simulink model "gm_ModeS_ADI_Codegen"  (R2017a)
settings: Solver=VariableStepDiscrete  StartTime=0.0  StopTime=1e6  RelTol=1e-3
PreLoadFcn:
  | load data_Yb;
  | 
  | DataIn = Yb_with_time(:,2);
  | 
  | wl=16;
undefined symbols (not defined in the file or in its folder): dfilt
libraries: simulink x3, dspobslib x2, dspsnks4 x2, hdlsllib x1, dspindex x1, dspsrcs4 x1
settings Model: Creator=mdonovan  LastModifiedBy=ACozma
settings DataIOCC: LimitDataPoints=on  SaveFormat=Array  SignalLoggingSaveFormat=ModelDataLogs  SaveOutput=off  SignalLogging=off  SaveTime=off
settings OptimizationCC: BlockReduction=off  BooleanDataType=off  ConditionallyExecuteInputs=off  DefaultParameterBehavior=Inlined  ExpressionDepthLimit=2147483647  LocalBlockOutputs=off  LifeSpan=inf
settings DebuggingCC: AlgebraicLoopMsg=error  UnderspecifiedInitializationDetection=Classic  MergeDetectMultiDrivingBlocksExec=none  SolverPrmCheckMsg=warning  InheritedTsInSrcMsg=none  SingleTaskRateTransMsg=error  FcnCallInpInsideContextMsg=warning  AllowSymbolicDim=off  StateNameClashWarn=warning  SFUnexpectedBacktrackingDiag=warning  SFNoUnconditionalDefaultTransitionDiag=warning  SFExecutionAtInitializationDiag=none
settings HardwareCC: ProdBitPerPointer=32  ProdBitPerSizeT=32  ProdBitPerPtrDiffT=32  ProdLargestAtomicFloat=None  ProdIntDivRoundTo=Undefined  ProdEndianess=Unspecified  ProdWordSize=32  ProdHWDeviceType=ASIC/FPGA->ASIC/FPGA  TargetBitPerPointer=64  TargetBitPerSizeT=64  TargetBitPerPtrDiffT=64  TargetLongLongMode=on  TargetIntDivRoundTo=Zero  TargetEndianess=LittleEndian  TargetWordSize=64  TargetHWDeviceType=MATLAB Host  ProdEqTarget=off
settings ModelReferenceCC: PropagateSignalLabelsOutOfModel=off
settings GRTTargetCC: TargetLangStandard=C89/C90 (ANSI)  GeneratePreprocessorConditionals=Disable all  CombineOutputUpdateFcns=off  GRTInterface=on
settings ConfigComp: CovMetricSettings=dw  CovHtmlReporting=on  CovSaveCumulativeToWorkspaceVar=on  CovSaveSingleToWorkspaceVar=on  CovExternalEMLEnable=off

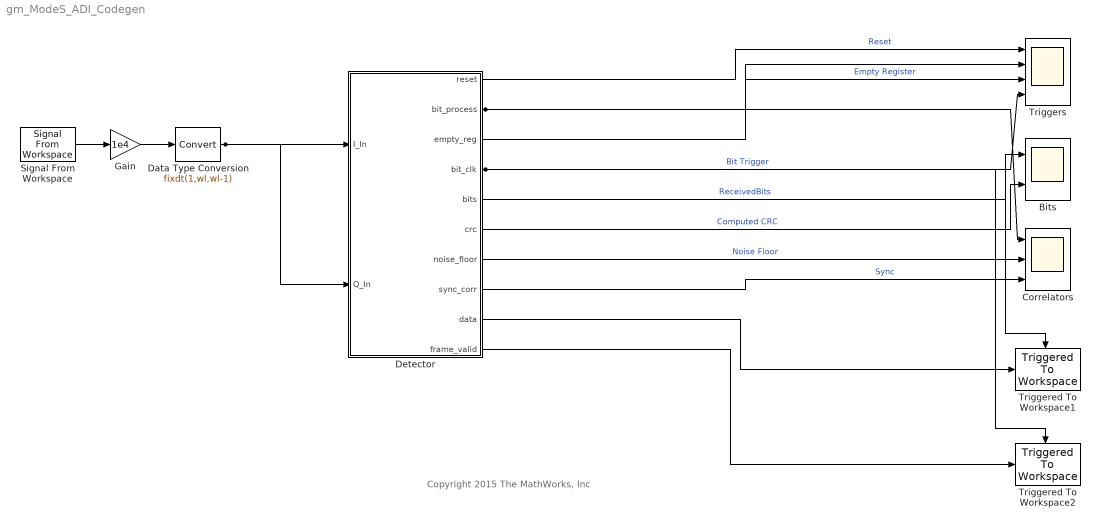
== system gm_ModeS_ADI_Codegen ==
  note: Copyright 2015 The MathWorks, Inc
  Bits : Scope  NumInputPorts=2
  Correlators : Scope  NumInputPorts=3
  Data Type Conversion : DataTypeConversion  OutDataTypeStr=fixdt(1,wl,wl-1)  LockScale=on
  Detector : Subsystem  TreatAsAtomicUnit=on
  Gain : Gain  Gain=1e4
  Signal From Workspace : dspsrcs4/Signal From Workspace  X=DataIn  Ts=1  nsamps=1  OutputAfterFinalValue=Setting to zero  ignoreOrWarnInputAndFrameLengths=off  OutputFrames=on
  Triggered To Workspace1 : dspsnks4/Triggered To Workspace  TriggerType=Rising edge  VariableName=data_out  Buffer=1000  Save2DMode=2-D array (concatenate along first dimension)
      settings: SourceProductName=DSP System Toolbox  SourceProductBaseCode=DS  FixptAsFi=off
  Triggered To Workspace2 : dspsnks4/Triggered To Workspace  TriggerType=Rising edge  VariableName=frame_valid  Buffer=1000  Save2DMode=2-D array (concatenate along first dimension)
      settings: SourceProductName=DSP System Toolbox  SourceProductBaseCode=DS  FixptAsFi=off
  Triggers : Scope  NumInputPorts=4
  wires:
  Detector/8(sync_corr) -> Correlators/3  "Sync"
  Detector/3(empty_reg) -> Triggers/3  "Empty Register"
  Detector/2(bit_process) -> Correlators/1, Triggers/2
  Detector/1(reset) -> Triggers/1  "Reset"
  Detector/6(crc) -> Bits/2  "Computed CRC"
  Detector/7(noise_floor) -> Correlators/2  "Noise Floor"
  Detector/9(data) -> Triggered To Workspace1/1
  Detector/10(frame_valid) -> Triggered To Workspace2/1
  Detector/4(bit_clk) -> Triggers/4, Triggered To Workspace1/Trigger, Triggered To Workspace2/Trigger  "Bit Trigger"
  Detector/5(bits) -> Bits/1  "ReceivedBits"
  Gain/1 -> Data Type Conversion/1
  Data Type Conversion/1 -> Detector/2(Q_In), Detector/1(I_In)
  Signal From Workspace/1 -> Gain/1

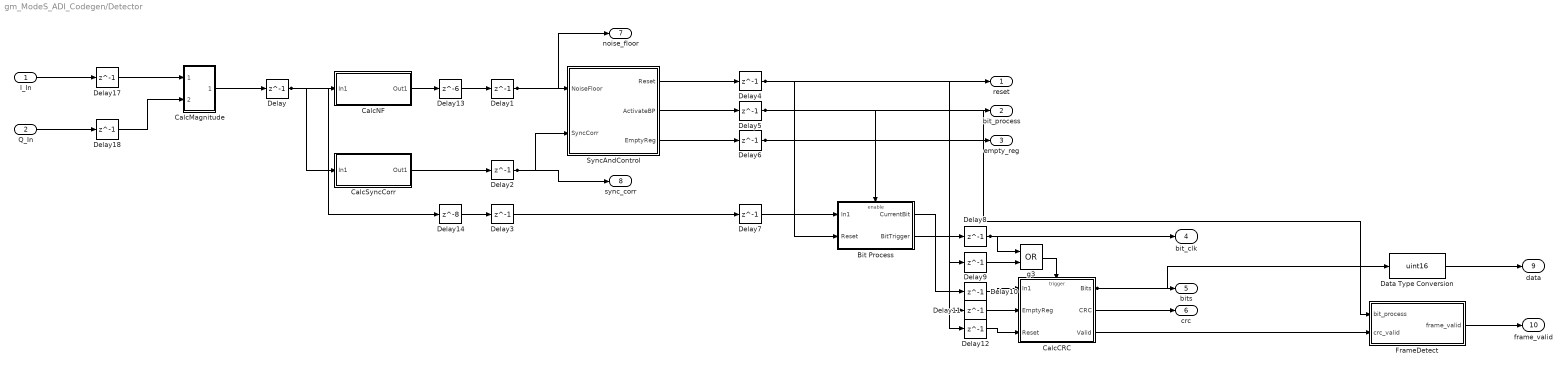
== system gm_ModeS_ADI_Codegen/Detector ==
  I_In : Inport  OutDataTypeStr=fixdt(1, 16, 15)  SampleTime=1
  Q_In : Inport  Port=2  OutDataTypeStr=fixdt(1, 16, 15)  SampleTime=1
  Bit Process : Subsystem
  CalcCRC : Subsystem
  CalcMagnitude : Subsystem
  CalcNF : Subsystem
  CalcSyncCorr : Subsystem
  Data Type Conversion : DataTypeConversion  OutDataTypeStr=uint16
  Delay{,1..12,17..18} (15 alike) : Delay  DelayLength=1  InitialCondition=0  InputProcessing=Columns as channels (frame based)
  Delay13 : Delay  DelayLength=6  InitialCondition=0  InputProcessing=Columns as channels (frame based)
  Delay14 : Delay  DelayLength=8  InitialCondition=0  InputProcessing=Columns as channels (frame based)
  FrameDetect : Subsystem
  SyncAndControl : Subsystem
  g3 : Logic  Operator=OR  AllPortsSameDT=off  OutDataTypeStr=boolean
  reset : Outport
  bit_process : Outport  Port=2
  empty_reg : Outport  Port=3
  bit_clk : Outport  Port=4
  bits : Outport  Port=5
  crc : Outport  Port=6
  noise_floor : Outport  Port=7
  sync_corr : Outport  Port=8
  data : Outport  Port=9
  frame_valid : Outport  Port=10
  wires:
  I_In/1 -> Delay17/1
  Q_In/1 -> Delay18/1
  Bit Process/1(CurrentBit) -> Delay10/1
  Bit Process/2(BitTrigger) -> Delay8/1
  CalcCRC/1(Bits) -> Data Type Conversion/1, bits/1
  CalcCRC/2(CRC) -> crc/1
  CalcCRC/3(Valid) -> FrameDetect/2(crc_valid)
  CalcMagnitude/1(Out1) -> Delay/1
  CalcNF/1(Out1) -> Delay13/1
  CalcSyncCorr/1(Out1) -> Delay2/1
  Data Type Conversion/1 -> data/1
  Delay/1 -> Delay14/1, CalcNF/1(In1), CalcSyncCorr/1(In1)
  Delay1/1 -> SyncAndControl/1(NoiseFloor), noise_floor/1
  Delay10/1 -> CalcCRC/1(In1)
  Delay11/1 -> CalcCRC/2(EmptyReg)
  Delay12/1 -> CalcCRC/3(Reset)
  Delay13/1 -> Delay1/1
  Delay14/1 -> Delay3/1
  Delay17/1 -> CalcMagnitude/1(In1)
  Delay18/1 -> CalcMagnitude/2(In2)
  Delay2/1 -> SyncAndControl/2(SyncCorr), sync_corr/1
  Delay3/1 -> Delay7/1
  Delay4/1 -> Delay9/1, Delay12/1, reset/1, Bit Process/2(Reset)
  Delay5/1 -> FrameDetect/1(bit_process), Bit Process/Enable, bit_process/1
  Delay6/1 -> Delay11/1, empty_reg/1
  Delay7/1 -> Bit Process/1(In1)
  Delay8/1 -> g3/1, bit_clk/1
  Delay9/1 -> g3/2
  FrameDetect/1(frame_valid) -> frame_valid/1
  SyncAndControl/1(Reset) -> Delay4/1
  SyncAndControl/2(ActivateBP) -> Delay5/1
  SyncAndControl/3(EmptyReg) -> Delay6/1
  g3/1 -> CalcCRC/Trigger

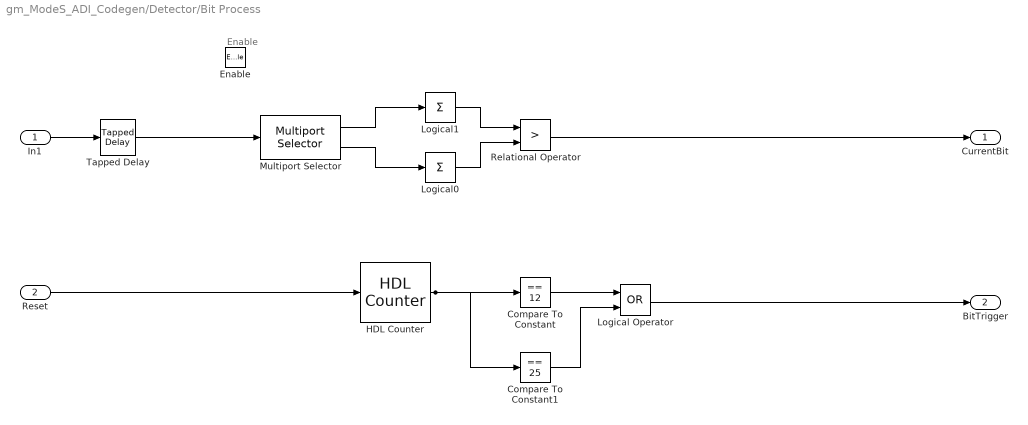
== system gm_ModeS_ADI_Codegen/Detector/Bit Process ==
  note: Enable
  In1 : Inport  SampleTime=1
  Reset : Inport  Port=2  SampleTime=1
  Enable : EnablePort
  Compare To Constant : simulink/Logic and Bit Operations/Compare To Constant  relop===  const=12  OutDataTypeStr=boolean
  Compare To Constant1 : simulink/Logic and Bit Operations/Compare To Constant  relop===  const=25  OutDataTypeStr=boolean
  HDL Counter : hdlsllib/HDL Operations/HDL Counter  CountType=Count limited  CountInit=1  CountStep=1  CountMax=25  CountFromType=Initial value  CountFrom=1  CountResetPort=on  CountLoadPort=off  CountEnbPort=off  CountDirPort=off  CountDataType=Unsigned  CountWordLen=8  CountFracLen=0  CountSampTime=1
      settings: SourceProductName=HDL Coder  SourceProductBaseCode=HD
  Logical Operator : Logic  Operator=OR  AllPortsSameDT=off  OutDataTypeStr=boolean
  Logical0 : Sum  Inputs=+  AccumDataTypeStr=fixdt(1,wl,wl-3)  OutDataTypeStr=Inherit: Same as accumulator
  Logical1 : Sum  Inputs=+  AccumDataTypeStr=fixdt(1,wl,wl-3)  OutDataTypeStr=Inherit: Same as accumulator
  Multiport Selector : dspindex/Multiport Selector  rowsOrCols=Rows  idxCellArray={ 1:6,7:12}  idxErrMode=Clip Index
  Relational Operator : RelationalOperator  Operator=>  OutDataTypeStr=boolean  RndMeth=Nearest
  Tapped Delay : simulink/Discrete/Tapped Delay  vinit=0.0  samptime=1  NumDelays=12  DelayOrder=Oldest  includeCurrent=on
  CurrentBit : Outport  InitialOutput=0
  BitTrigger : Outport  Port=2  InitialOutput=0
  wires:
  In1/1 -> Tapped Delay/1
  Reset/1 -> HDL Counter/1
  Compare To Constant/1 -> Logical Operator/1
  Compare To Constant1/1 -> Logical Operator/2
  HDL Counter/1 -> Compare To Constant1/1, Compare To Constant/1
  Logical Operator/1 -> BitTrigger/1
  Logical0/1 -> Relational Operator/2
  Logical1/1 -> Relational Operator/1
  Multiport Selector/1 -> Logical1/1
  Multiport Selector/2 -> Logical0/1
  Relational Operator/1 -> CurrentBit/1
  Tapped Delay/1 -> Multiport Selector/1

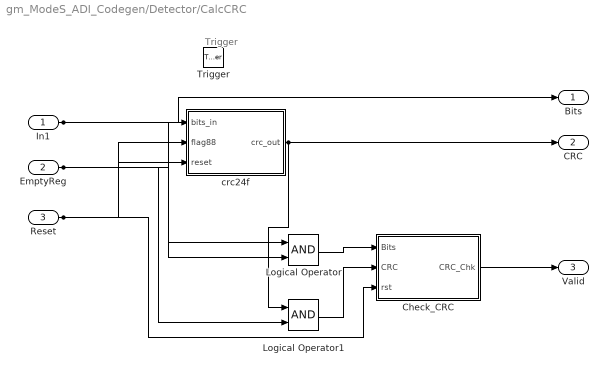
== system gm_ModeS_ADI_Codegen/Detector/CalcCRC ==
  note: Trigger
  In1 : Inport
  EmptyReg : Inport  Port=2
  Reset : Inport  Port=3
  Trigger : TriggerPort  VariantControl=Variant
  Check_CRC : Subsystem
  Logical Operator : Logic  AllPortsSameDT=off  OutDataTypeStr=boolean
  Logical Operator1 : Logic  AllPortsSameDT=off  OutDataTypeStr=boolean
  crc24f : Subsystem
  Bits : Outport  InitialOutput=0
  CRC : Outport  Port=2  InitialOutput=0
  Valid : Outport  Port=3  InitialOutput=0
  wires:
  In1/1 -> Logical Operator/1, Bits/1, crc24f/1(bits_in)
  EmptyReg/1 -> Logical Operator1/2, Logical Operator/2, crc24f/2(flag88)
  Reset/1 -> Check_CRC/3(rst), crc24f/3(reset)
  Check_CRC/1(CRC_Chk) -> Valid/1
  Logical Operator/1 -> Check_CRC/1(Bits)
  Logical Operator1/1 -> Check_CRC/2(CRC)
  crc24f/1(crc_out) -> Logical Operator1/1, CRC/1

== system gm_ModeS_ADI_Codegen/Detector/CalcMagnitude ==
  In1 : Inport  SampleTime=1
  In2 : Inport  Port=2  SampleTime=1
  Add : Sum  OutDataTypeStr=fixdt(1,wl,wl-1)
  Delay15 : Delay  DelayLength=1  InitialCondition=0  InputProcessing=Columns as channels (frame based)
  Delay16 : Delay  DelayLength=1  InitialCondition=0  InputProcessing=Columns as channels (frame based)
  Product : Product  OutDataTypeStr=fixdt(1,wl,wl-1)
  Product1 : Product  OutDataTypeStr=fixdt(1,wl,wl-1)
  Out1 : Outport
  wires:
  In1/1 -> Product/2, Product/1
  In2/1 -> Product1/2, Product1/1
  Add/1 -> Out1/1
  Delay15/1 -> Add/1
  Delay16/1 -> Add/2
  Product/1 -> Delay15/1
  Product1/1 -> Delay16/1

== system gm_ModeS_ADI_Codegen/Detector/CalcNF ==
  In1 : Inport  SampleTime=1
  NoiseFloor : Subsystem
      settings: DeleteFcn=dspLinkFVTool2Mask(gcbh,'close')  ModelCloseFcn=dspLinkFVTool2Mask(gcbh,'close')  CloseFcn=dspLinkFVTool2Mask(gcbh,'close')
  Out1 : Outport
  wires:
  In1/1 -> NoiseFloor/1(In1)
  NoiseFloor/1(Out1) -> Out1/1

== system gm_ModeS_ADI_Codegen/Detector/CalcSyncCorr ==
  In1 : Inport  SampleTime=1
  SyncCorr : Subsystem
      settings: DeleteFcn=dspLinkFVTool2Mask(gcbh,'close')  ModelCloseFcn=dspLinkFVTool2Mask(gcbh,'close')  CloseFcn=dspLinkFVTool2Mask(gcbh,'close')
  Out1 : Outport
  wires:
  In1/1 -> SyncCorr/1(In1)
  SyncCorr/1(Out1) -> Out1/1

== system gm_ModeS_ADI_Codegen/Detector/FrameDetect ==
  bit_process : Inport  SampleTime=1
  crc_valid : Inport  Port=2  SampleTime=1
  Data Type Conversion : DataTypeConversion  OutDataTypeStr=uint16
  Delay14 : Delay  DelayLength=1  InitialCondition=0  InputProcessing=Columns as channels (frame based)
  Logical Operator : Logic  AllPortsSameDT=off  OutDataTypeStr=boolean
  Logical Operator1 : Logic  Operator=NOT  AllPortsSameDT=off  OutDataTypeStr=boolean
  Logical Operator2 : Logic  AllPortsSameDT=off  OutDataTypeStr=boolean
  frame_valid : Outport
  wires:
  bit_process/1 -> Logical Operator1/1, Delay14/1
  crc_valid/1 -> Logical Operator2/1
  Data Type Conversion/1 -> frame_valid/1
  Delay14/1 -> Logical Operator/2
  Logical Operator/1 -> Logical Operator2/2
  Logical Operator1/1 -> Logical Operator/1
  Logical Operator2/1 -> Data Type Conversion/1

== system gm_ModeS_ADI_Codegen/Detector/SyncAndControl ==
  NoiseFloor : Inport  SampleTime=1
  SyncCorr : Inport  Port=2  SampleTime=1
  SyncAndControl : Stateflow chart  TreatAsAtomicUnit=on
  Reset : Outport
  ActivateBP : Outport  Port=2
  EmptyReg : Outport  Port=3
  wires:
  NoiseFloor/1 -> SyncAndControl/1(NoiseFloor)
  SyncCorr/1 -> SyncAndControl/2(SyncCorr)
  SyncAndControl/1(Reset) -> Reset/1
  SyncAndControl/2(ActivateBP) -> ActivateBP/1
  SyncAndControl/3(EmptyReg) -> EmptyReg/1

== system gm_ModeS_ADI_Codegen/Detector/CalcCRC/Check_CRC ==
  note: Remember any difference
  note: Comparison
  Bits : Inport
  CRC : Inport  Port=2
  rst : Inport  Port=3
  Delay : Delay  DelayLength=1  ExternalReset=Level
      settings: InputPortMap=u0,r5
  Logical Operator : Logic  Operator=XOR  AllPortsSameDT=off  OutDataTypeStr=boolean
  Logical Operator1 : Logic  Operator=OR  AllPortsSameDT=off  OutDataTypeStr=boolean
  Logical Operator2 : Logic  Operator=NOT  AllPortsSameDT=off  OutDataTypeStr=boolean
  CRC_Chk : Outport  InitialOutput=0
  wires:
  Bits/1 -> Logical Operator/1
  CRC/1 -> Logical Operator/2
  rst/1 -> Delay/2
  Logical Operator/1 -> Logical Operator1/1
  Logical Operator1/1 -> Logical Operator2/1, Delay/1
  Logical Operator2/1 -> CRC_Chk/1
  Delay/1 -> Logical Operator1/2

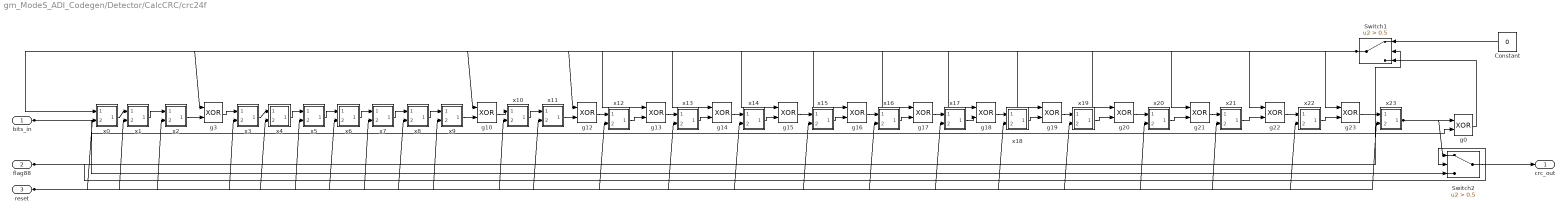
== system gm_ModeS_ADI_Codegen/Detector/CalcCRC/crc24f ==
  bits_in : Inport
  flag88 : Inport  Port=2
  reset : Inport  Port=3
  Constant : Constant  Value=0  OutDataTypeStr=boolean  SampleTime=-1
  Switch1 : Switch  Criteria=u2 > Threshold  Threshold=0.5
  Switch2 : Switch  Criteria=u2 > Threshold  Threshold=0.5
  g{0,3,10,12..23} (15 alike) : Logic  Operator=XOR  AllPortsSameDT=off  OutDataTypeStr=boolean
  x0 : Subsystem
  x1 : Subsystem
  x10 : Subsystem
  x11 : Subsystem
  x12 : Subsystem
  x13 : Subsystem
  x14 : Subsystem
  x15 : Subsystem
  x16 : Subsystem
  x17 : Subsystem
  x18 : Subsystem
  x19 : Subsystem
  x2 : Subsystem
  x20 : Subsystem
  x21 : Subsystem
  x22 : Subsystem
  x23 : Subsystem
  x3 : Subsystem
  x4 : Subsystem
  x5 : Subsystem
  x6 : Subsystem
  x7 : Subsystem
  x8 : Subsystem
  x9 : Subsystem
  crc_out : Outport  InitialOutput=0
  wires:
  bits_in/1 -> Switch2/3, g0/2
  flag88/1 -> Switch2/2, Switch1/2
  reset/1 -> x0/2(Reset), x1/2(Reset), x10/2(Reset), x11/2(Reset), x12/2(Reset), x13/2(Reset), x14/2(Reset), x15/2(Reset), x16/2(Reset), x17/2(Reset), x18/2(Reset), x19/2(Reset), x2/2(Reset), x20/2(Reset), x21/2(Reset), x22/2(Reset), x23/2(Reset), x3/2(Reset), x4/2(Reset), x5/2(Reset), x6/2(Reset), x7/2(Reset), x8/2(Reset), x9/2(Reset)
  Constant/1 -> Switch1/1
  Switch2/1 -> crc_out/1
  x23/1(data_out) -> Switch2/1, g0/1
  x22/1(data_out) -> g23/2
  g22/1 -> x22/1(data_in)
  x21/1(data_out) -> g22/2
  g21/1 -> x21/1(data_in)
  x20/1(data_out) -> g21/2
  g20/1 -> x20/1(data_in)
  x19/1(data_out) -> g20/2
  g19/1 -> x19/1(data_in)
  x18/1(data_out) -> g19/2
  g18/1 -> x18/1(data_in)
  x17/1(data_out) -> g18/2
  g17/1 -> x17/1(data_in)
  x16/1(data_out) -> g17/2
  g16/1 -> x16/1(data_in)
  x15/1(data_out) -> g16/2
  g15/1 -> x15/1(data_in)
  x14/1(data_out) -> g15/2
  g14/1 -> x14/1(data_in)
  x13/1(data_out) -> g14/2
  g13/1 -> x13/1(data_in)
  x12/1(data_out) -> g13/2
  g12/1 -> x12/1(data_in)
  x11/1(data_out) -> g12/2
  x10/1(data_out) -> x11/1(data_in)
  g10/1 -> x10/1(data_in)
  x9/1(data_out) -> g10/2
  x8/1(data_out) -> x9/1(data_in)
  x7/1(data_out) -> x8/1(data_in)
  x6/1(data_out) -> x7/1(data_in)
  x5/1(data_out) -> x6/1(data_in)
  x4/1(data_out) -> x5/1(data_in)
  x3/1(data_out) -> x4/1(data_in)
  g3/1 -> x3/1(data_in)
  x2/1(data_out) -> g3/2
  x1/1(data_out) -> x2/1(data_in)
  x0/1(data_out) -> x1/1(data_in)
  g0/1 -> Switch1/3
  Switch1/1 -> g3/1, g23/1, g22/1, g21/1, g20/1, g19/1, g18/1, g17/1, g16/1, g15/1, g14/1, g13/1, g12/1, g10/1, x0/1(data_in)
  g23/1 -> x23/1(data_in)

== system gm_ModeS_ADI_Codegen/Detector/CalcNF/NoiseFloor ==
  In1 : Inport
  NoiseFloor : dspobslib/Digital Filter  TypePopup=FIR (all zeros)  IIRFiltStruct=Direct form II transposed  AllPoleFiltStruct=Direct form  FIRFiltStruct=Direct form transposed  CoeffSource=Specify via dialog  NumCoeffs=(ones(64,1)/64)  DenCoeffs=[1 0.1]  BiQuadCoeffs=[1 0.3 0.4 1 0.1 0.2]  LatticeCoeffs=[0.2 0.4]  denIgnore=on  FiltPerSampPopup=One filter per frame  IC=0  ICnum=0  ICden=0  firstCoeffMode=Binary point scaling  firstCoeffWordLength=wl  firstCoeffFracLength=wl+4  outputMode=Binary point scaling  outputWordLength=wl  outputFracLength=wl  accumMode=Binary point scaling  accumWordLength=wl*2  accumFracLength=wl*2  prodOutputMode=Binary point scaling  prodOutputWordLength=wl*2  prodOutputFracLength=wl*2+5  roundingMode=Floor  overflowMode=off  ScaleValues=1  scaleValueFracLength=14  stageInFracLength=15  stageOutFracLength=15  FilterSource=Specify via dialog  dfiltObjectName=dfilt.dffir([1 2 1])  InputProcessing=Columns as channels (frame based)
      settings: SourceProductName=DSP System Toolbox  SourceProductBaseCode=DS
  NoiseFloor_GenDelay1 : Delay  InputProcessing=Inherited
  Out1 : Outport
  wires:
  In1/1 -> NoiseFloor/1
  NoiseFloor/1 -> NoiseFloor_GenDelay1/1
  NoiseFloor_GenDelay1/1 -> Out1/1

== system gm_ModeS_ADI_Codegen/Detector/CalcSyncCorr/SyncCorr ==
  In1 : Inport
  SyncCorr : dspobslib/Digital Filter  TypePopup=FIR (all zeros)  IIRFiltStruct=Direct form II transposed  AllPoleFiltStruct=Direct form  FIRFiltStruct=Direct form  CoeffSource=Specify via dialog  NumCoeffs=|  DenCoeffs=[1 0.1]  BiQuadCoeffs=[1 0.3 0.4 1 0.1 0.2]  LatticeCoeffs=[0.2 0.4]  denIgnore=on  FiltPerSampPopup=One filter per frame  IC=0  ICnum=0  ICden=0  firstCoeffMode=Binary point scaling  firstCoeffWordLength=16  firstCoeffFracLength=14  outputMode=Binary point scaling  outputWordLength=16  outputFracLength=11  accumMode=Binary point scaling  accumWordLength=37  accumFracLength=29  prodOutputMode=Binary point scaling  prodOutputWordLength=31  prodOutputFracLength=29  roundingMode=Floor  overflowMode=off  ScaleValues=1  scaleValueFracLength=14  stageInFracLength=15  stageOutFracLength=15  FilterSource=Specify via dialog  dfiltObjectName=dfilt.dffir([1 2 1])  InputProcessing=Columns as channels (frame based)
      | flipud([ones(6,1);-1*ones(6,1);ones(6,1);-1*ones(7,1);
      | -1*ones(6,1);-1*ones(6,1);-1*ones(6,1);ones(7,1);-1*ones(6,1);ones(6,1);-1*ones(6,1);-1*ones(7,1)])
      settings: SourceProductName=DSP System Toolbox  SourceProductBaseCode=DS
  SyncCorr_GenDelay1 : Delay  DelayLength=8  InputProcessing=Inherited
  Out1 : Outport
  wires:
  In1/1 -> SyncCorr/1
  SyncCorr/1 -> SyncCorr_GenDelay1/1
  SyncCorr_GenDelay1/1 -> Out1/1

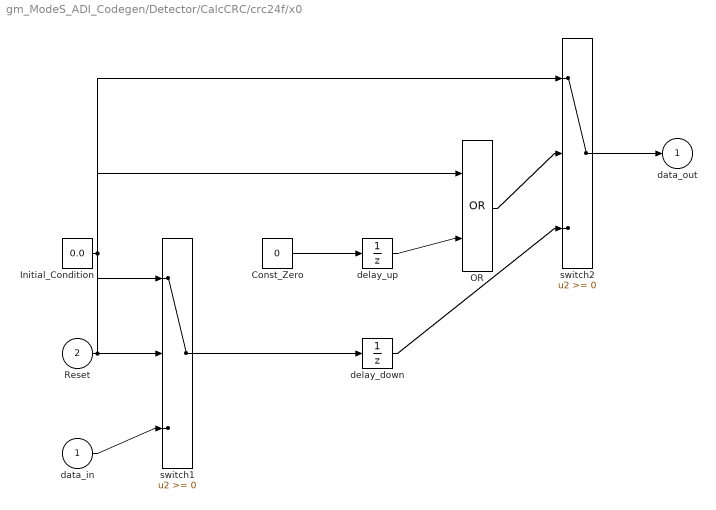
== system gm_ModeS_ADI_Codegen/Detector/CalcCRC/crc24f/x0 ==
  data_in : Inport
  Reset : Inport  Port=2
  Const_Zero : Constant  Value=0  OutDataTypeStr=boolean
  Initial_Condition : Constant  Value=0.0  OutDataTypeStr=Inherit: Inherit via back propagation
  OR : Logic  Operator=OR
  delay_down : UnitDelay  SampleTime=-1
  delay_up : UnitDelay  InitialCondition=1  SampleTime=-1
  switch1 : Switch  SaturateOnIntegerOverflow=on  InputSameDT=on
  switch2 : Switch  SaturateOnIntegerOverflow=on  InputSameDT=on
  data_out : Outport
  wires:
  Initial_Condition/1 -> switch1/1, switch2/1
  Reset/1 -> switch1/2, OR/1
  data_in/1 -> switch1/3
  Const_Zero/1 -> delay_up/1
  switch1/1 -> delay_down/1
  delay_up/1 -> OR/2
  OR/1 -> switch2/2
  delay_down/1 -> switch2/3
  switch2/1 -> data_out/1

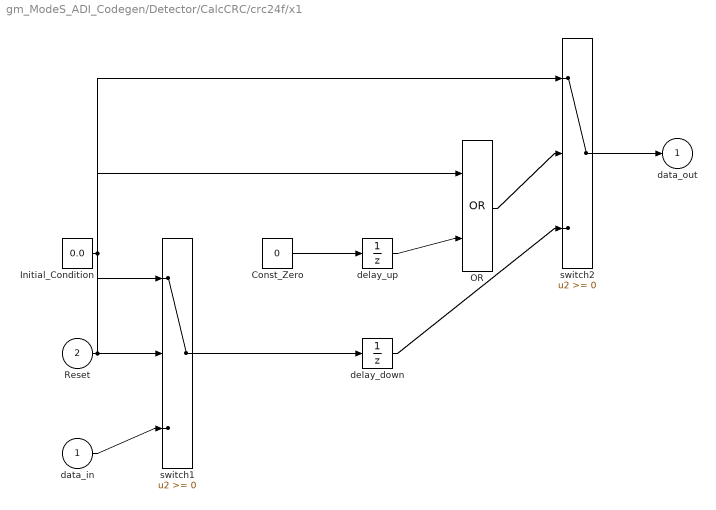
== system gm_ModeS_ADI_Codegen/Detector/CalcCRC/crc24f/x1 ==
  data_in : Inport
  Reset : Inport  Port=2
  Const_Zero : Constant  Value=0  OutDataTypeStr=boolean
  Initial_Condition : Constant  Value=0.0  OutDataTypeStr=Inherit: Inherit via back propagation
  OR : Logic  Operator=OR
  delay_down : UnitDelay  SampleTime=-1
  delay_up : UnitDelay  InitialCondition=1  SampleTime=-1
  switch1 : Switch  SaturateOnIntegerOverflow=on  InputSameDT=on
  switch2 : Switch  SaturateOnIntegerOverflow=on  InputSameDT=on
  data_out : Outport
  wires:
  Initial_Condition/1 -> switch1/1, switch2/1
  Reset/1 -> switch1/2, OR/1
  data_in/1 -> switch1/3
  Const_Zero/1 -> delay_up/1
  switch1/1 -> delay_down/1
  delay_up/1 -> OR/2
  OR/1 -> switch2/2
  delay_down/1 -> switch2/3
  switch2/1 -> data_out/1

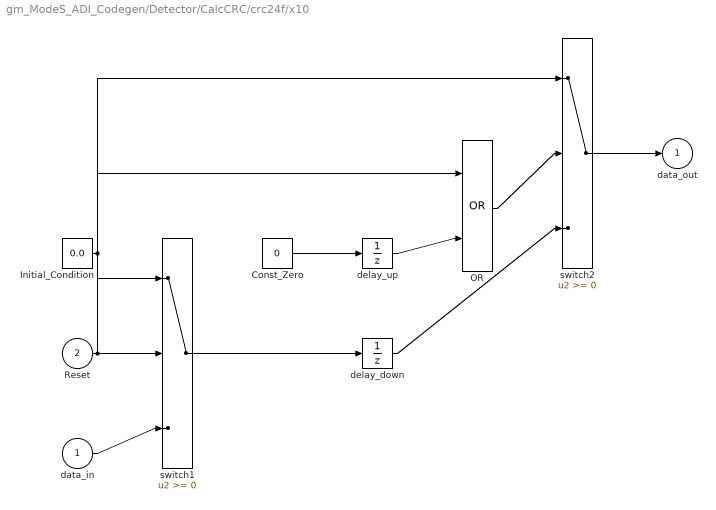
== system gm_ModeS_ADI_Codegen/Detector/CalcCRC/crc24f/x10 ==
  data_in : Inport
  Reset : Inport  Port=2
  Const_Zero : Constant  Value=0  OutDataTypeStr=boolean
  Initial_Condition : Constant  Value=0.0  OutDataTypeStr=Inherit: Inherit via back propagation
  OR : Logic  Operator=OR
  delay_down : UnitDelay  SampleTime=-1
  delay_up : UnitDelay  InitialCondition=1  SampleTime=-1
  switch1 : Switch  SaturateOnIntegerOverflow=on  InputSameDT=on
  switch2 : Switch  SaturateOnIntegerOverflow=on  InputSameDT=on
  data_out : Outport
  wires:
  Initial_Condition/1 -> switch1/1, switch2/1
  Reset/1 -> switch1/2, OR/1
  data_in/1 -> switch1/3
  Const_Zero/1 -> delay_up/1
  switch1/1 -> delay_down/1
  delay_up/1 -> OR/2
  OR/1 -> switch2/2
  delay_down/1 -> switch2/3
  switch2/1 -> data_out/1

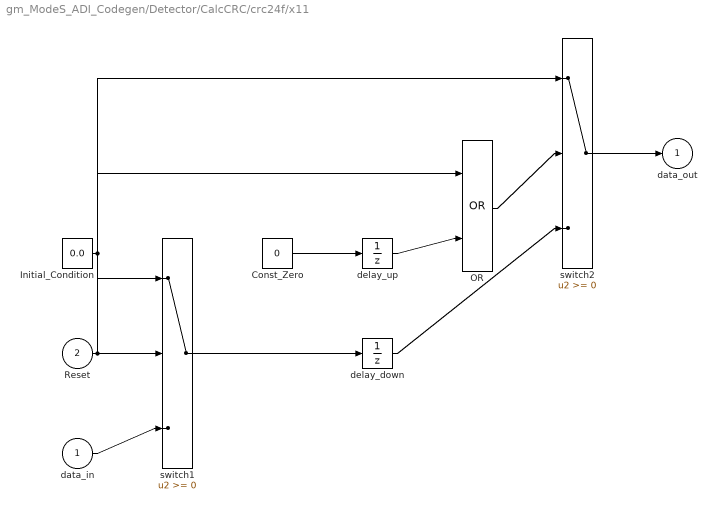
== system gm_ModeS_ADI_Codegen/Detector/CalcCRC/crc24f/x11 ==
  data_in : Inport
  Reset : Inport  Port=2
  Const_Zero : Constant  Value=0  OutDataTypeStr=boolean
  Initial_Condition : Constant  Value=0.0  OutDataTypeStr=Inherit: Inherit via back propagation
  OR : Logic  Operator=OR
  delay_down : UnitDelay  SampleTime=-1
  delay_up : UnitDelay  InitialCondition=1  SampleTime=-1
  switch1 : Switch  SaturateOnIntegerOverflow=on  InputSameDT=on
  switch2 : Switch  SaturateOnIntegerOverflow=on  InputSameDT=on
  data_out : Outport
  wires:
  Initial_Condition/1 -> switch1/1, switch2/1
  Reset/1 -> switch1/2, OR/1
  data_in/1 -> switch1/3
  Const_Zero/1 -> delay_up/1
  switch1/1 -> delay_down/1
  delay_up/1 -> OR/2
  OR/1 -> switch2/2
  delay_down/1 -> switch2/3
  switch2/1 -> data_out/1

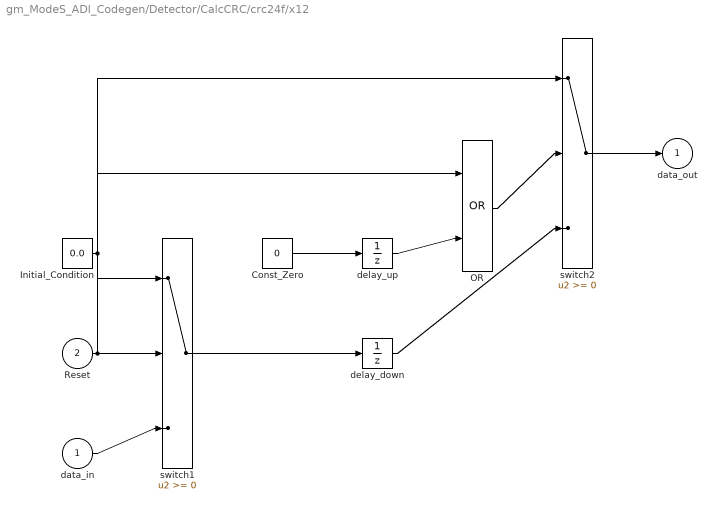
== system gm_ModeS_ADI_Codegen/Detector/CalcCRC/crc24f/x12 ==
  data_in : Inport
  Reset : Inport  Port=2
  Const_Zero : Constant  Value=0  OutDataTypeStr=boolean
  Initial_Condition : Constant  Value=0.0  OutDataTypeStr=Inherit: Inherit via back propagation
  OR : Logic  Operator=OR
  delay_down : UnitDelay  SampleTime=-1
  delay_up : UnitDelay  InitialCondition=1  SampleTime=-1
  switch1 : Switch  SaturateOnIntegerOverflow=on  InputSameDT=on
  switch2 : Switch  SaturateOnIntegerOverflow=on  InputSameDT=on
  data_out : Outport
  wires:
  Initial_Condition/1 -> switch1/1, switch2/1
  Reset/1 -> switch1/2, OR/1
  data_in/1 -> switch1/3
  Const_Zero/1 -> delay_up/1
  switch1/1 -> delay_down/1
  delay_up/1 -> OR/2
  OR/1 -> switch2/2
  delay_down/1 -> switch2/3
  switch2/1 -> data_out/1

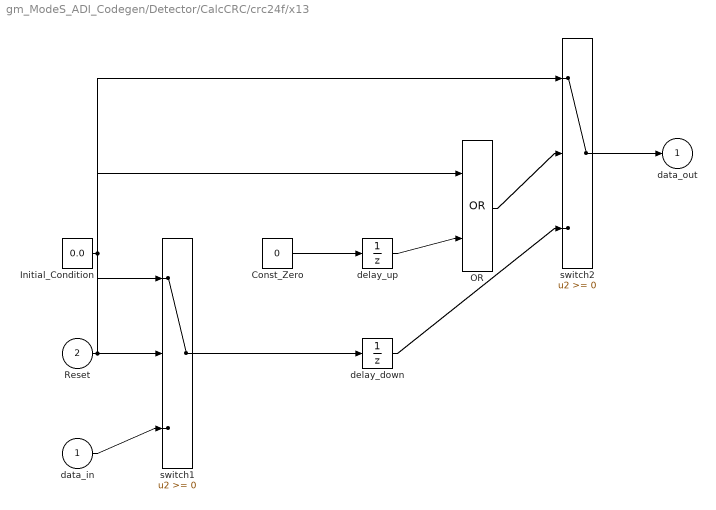
== system gm_ModeS_ADI_Codegen/Detector/CalcCRC/crc24f/x13 ==
  data_in : Inport
  Reset : Inport  Port=2
  Const_Zero : Constant  Value=0  OutDataTypeStr=boolean
  Initial_Condition : Constant  Value=0.0  OutDataTypeStr=Inherit: Inherit via back propagation
  OR : Logic  Operator=OR
  delay_down : UnitDelay  SampleTime=-1
  delay_up : UnitDelay  InitialCondition=1  SampleTime=-1
  switch1 : Switch  SaturateOnIntegerOverflow=on  InputSameDT=on
  switch2 : Switch  SaturateOnIntegerOverflow=on  InputSameDT=on
  data_out : Outport
  wires:
  Initial_Condition/1 -> switch1/1, switch2/1
  Reset/1 -> switch1/2, OR/1
  data_in/1 -> switch1/3
  Const_Zero/1 -> delay_up/1
  switch1/1 -> delay_down/1
  delay_up/1 -> OR/2
  OR/1 -> switch2/2
  delay_down/1 -> switch2/3
  switch2/1 -> data_out/1

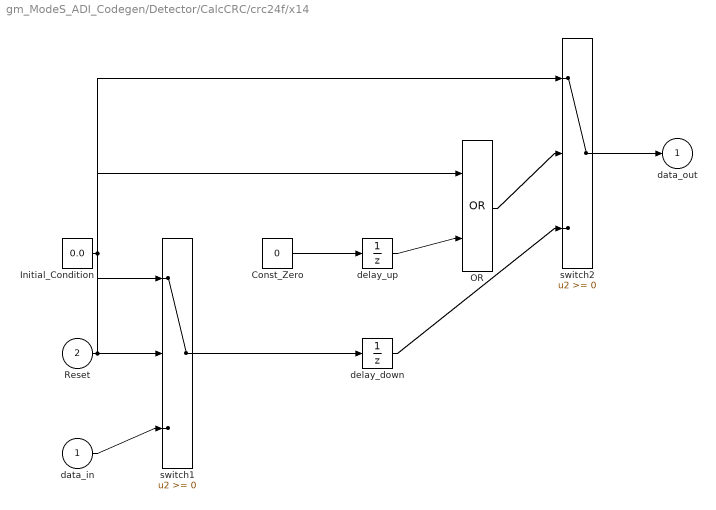
== system gm_ModeS_ADI_Codegen/Detector/CalcCRC/crc24f/x14 ==
  data_in : Inport
  Reset : Inport  Port=2
  Const_Zero : Constant  Value=0  OutDataTypeStr=boolean
  Initial_Condition : Constant  Value=0.0  OutDataTypeStr=Inherit: Inherit via back propagation
  OR : Logic  Operator=OR
  delay_down : UnitDelay  SampleTime=-1
  delay_up : UnitDelay  InitialCondition=1  SampleTime=-1
  switch1 : Switch  SaturateOnIntegerOverflow=on  InputSameDT=on
  switch2 : Switch  SaturateOnIntegerOverflow=on  InputSameDT=on
  data_out : Outport
  wires:
  Initial_Condition/1 -> switch1/1, switch2/1
  Reset/1 -> switch1/2, OR/1
  data_in/1 -> switch1/3
  Const_Zero/1 -> delay_up/1
  switch1/1 -> delay_down/1
  delay_up/1 -> OR/2
  OR/1 -> switch2/2
  delay_down/1 -> switch2/3
  switch2/1 -> data_out/1

== system gm_ModeS_ADI_Codegen/Detector/CalcCRC/crc24f/x15 ==
  data_in : Inport
  Reset : Inport  Port=2
  Const_Zero : Constant  Value=0  OutDataTypeStr=boolean
  Initial_Condition : Constant  Value=0.0  OutDataTypeStr=Inherit: Inherit via back propagation
  OR : Logic  Operator=OR
  delay_down : UnitDelay  SampleTime=-1
  delay_up : UnitDelay  InitialCondition=1  SampleTime=-1
  switch1 : Switch  SaturateOnIntegerOverflow=on  InputSameDT=on
  switch2 : Switch  SaturateOnIntegerOverflow=on  InputSameDT=on
  data_out : Outport
  wires:
  Initial_Condition/1 -> switch1/1, switch2/1
  Reset/1 -> switch1/2, OR/1
  data_in/1 -> switch1/3
  Const_Zero/1 -> delay_up/1
  switch1/1 -> delay_down/1
  delay_up/1 -> OR/2
  OR/1 -> switch2/2
  delay_down/1 -> switch2/3
  switch2/1 -> data_out/1

== system gm_ModeS_ADI_Codegen/Detector/CalcCRC/crc24f/x16 ==
  data_in : Inport
  Reset : Inport  Port=2
  Const_Zero : Constant  Value=0  OutDataTypeStr=boolean
  Initial_Condition : Constant  Value=0.0  OutDataTypeStr=Inherit: Inherit via back propagation
  OR : Logic  Operator=OR
  delay_down : UnitDelay  SampleTime=-1
  delay_up : UnitDelay  InitialCondition=1  SampleTime=-1
  switch1 : Switch  SaturateOnIntegerOverflow=on  InputSameDT=on
  switch2 : Switch  SaturateOnIntegerOverflow=on  InputSameDT=on
  data_out : Outport
  wires:
  Initial_Condition/1 -> switch1/1, switch2/1
  Reset/1 -> switch1/2, OR/1
  data_in/1 -> switch1/3
  Const_Zero/1 -> delay_up/1
  switch1/1 -> delay_down/1
  delay_up/1 -> OR/2
  OR/1 -> switch2/2
  delay_down/1 -> switch2/3
  switch2/1 -> data_out/1

== system gm_ModeS_ADI_Codegen/Detector/CalcCRC/crc24f/x17 ==
  data_in : Inport
  Reset : Inport  Port=2
  Const_Zero : Constant  Value=0  OutDataTypeStr=boolean
  Initial_Condition : Constant  Value=0.0  OutDataTypeStr=Inherit: Inherit via back propagation
  OR : Logic  Operator=OR
  delay_down : UnitDelay  SampleTime=-1
  delay_up : UnitDelay  InitialCondition=1  SampleTime=-1
  switch1 : Switch  SaturateOnIntegerOverflow=on  InputSameDT=on
  switch2 : Switch  SaturateOnIntegerOverflow=on  InputSameDT=on
  data_out : Outport
  wires:
  Initial_Condition/1 -> switch1/1, switch2/1
  Reset/1 -> switch1/2, OR/1
  data_in/1 -> switch1/3
  Const_Zero/1 -> delay_up/1
  switch1/1 -> delay_down/1
  delay_up/1 -> OR/2
  OR/1 -> switch2/2
  delay_down/1 -> switch2/3
  switch2/1 -> data_out/1

== system gm_ModeS_ADI_Codegen/Detector/CalcCRC/crc24f/x18 ==
  data_in : Inport
  Reset : Inport  Port=2
  Const_Zero : Constant  Value=0  OutDataTypeStr=boolean
  Initial_Condition : Constant  Value=0.0  OutDataTypeStr=Inherit: Inherit via back propagation
  OR : Logic  Operator=OR
  delay_down : UnitDelay  SampleTime=-1
  delay_up : UnitDelay  InitialCondition=1  SampleTime=-1
  switch1 : Switch  SaturateOnIntegerOverflow=on  InputSameDT=on
  switch2 : Switch  SaturateOnIntegerOverflow=on  InputSameDT=on
  data_out : Outport
  wires:
  Initial_Condition/1 -> switch1/1, switch2/1
  Reset/1 -> switch1/2, OR/1
  data_in/1 -> switch1/3
  Const_Zero/1 -> delay_up/1
  switch1/1 -> delay_down/1
  delay_up/1 -> OR/2
  OR/1 -> switch2/2
  delay_down/1 -> switch2/3
  switch2/1 -> data_out/1

== system gm_ModeS_ADI_Codegen/Detector/CalcCRC/crc24f/x19 ==
  data_in : Inport
  Reset : Inport  Port=2
  Const_Zero : Constant  Value=0  OutDataTypeStr=boolean
  Initial_Condition : Constant  Value=0.0  OutDataTypeStr=Inherit: Inherit via back propagation
  OR : Logic  Operator=OR
  delay_down : UnitDelay  SampleTime=-1
  delay_up : UnitDelay  InitialCondition=1  SampleTime=-1
  switch1 : Switch  SaturateOnIntegerOverflow=on  InputSameDT=on
  switch2 : Switch  SaturateOnIntegerOverflow=on  InputSameDT=on
  data_out : Outport
  wires:
  Initial_Condition/1 -> switch1/1, switch2/1
  Reset/1 -> switch1/2, OR/1
  data_in/1 -> switch1/3
  Const_Zero/1 -> delay_up/1
  switch1/1 -> delay_down/1
  delay_up/1 -> OR/2
  OR/1 -> switch2/2
  delay_down/1 -> switch2/3
  switch2/1 -> data_out/1

== system gm_ModeS_ADI_Codegen/Detector/CalcCRC/crc24f/x2 ==
  data_in : Inport
  Reset : Inport  Port=2
  Const_Zero : Constant  Value=0  OutDataTypeStr=boolean
  Initial_Condition : Constant  Value=0.0  OutDataTypeStr=Inherit: Inherit via back propagation
  OR : Logic  Operator=OR
  delay_down : UnitDelay  SampleTime=-1
  delay_up : UnitDelay  InitialCondition=1  SampleTime=-1
  switch1 : Switch  SaturateOnIntegerOverflow=on  InputSameDT=on
  switch2 : Switch  SaturateOnIntegerOverflow=on  InputSameDT=on
  data_out : Outport
  wires:
  Initial_Condition/1 -> switch1/1, switch2/1
  Reset/1 -> switch1/2, OR/1
  data_in/1 -> switch1/3
  Const_Zero/1 -> delay_up/1
  switch1/1 -> delay_down/1
  delay_up/1 -> OR/2
  OR/1 -> switch2/2
  delay_down/1 -> switch2/3
  switch2/1 -> data_out/1

== system gm_ModeS_ADI_Codegen/Detector/CalcCRC/crc24f/x20 ==
  data_in : Inport
  Reset : Inport  Port=2
  Const_Zero : Constant  Value=0  OutDataTypeStr=boolean
  Initial_Condition : Constant  Value=0.0  OutDataTypeStr=Inherit: Inherit via back propagation
  OR : Logic  Operator=OR
  delay_down : UnitDelay  SampleTime=-1
  delay_up : UnitDelay  InitialCondition=1  SampleTime=-1
  switch1 : Switch  SaturateOnIntegerOverflow=on  InputSameDT=on
  switch2 : Switch  SaturateOnIntegerOverflow=on  InputSameDT=on
  data_out : Outport
  wires:
  Initial_Condition/1 -> switch1/1, switch2/1
  Reset/1 -> switch1/2, OR/1
  data_in/1 -> switch1/3
  Const_Zero/1 -> delay_up/1
  switch1/1 -> delay_down/1
  delay_up/1 -> OR/2
  OR/1 -> switch2/2
  delay_down/1 -> switch2/3
  switch2/1 -> data_out/1

== system gm_ModeS_ADI_Codegen/Detector/CalcCRC/crc24f/x21 ==
  data_in : Inport
  Reset : Inport  Port=2
  Const_Zero : Constant  Value=0  OutDataTypeStr=boolean
  Initial_Condition : Constant  Value=0.0  OutDataTypeStr=Inherit: Inherit via back propagation
  OR : Logic  Operator=OR
  delay_down : UnitDelay  SampleTime=-1
  delay_up : UnitDelay  InitialCondition=1  SampleTime=-1
  switch1 : Switch  SaturateOnIntegerOverflow=on  InputSameDT=on
  switch2 : Switch  SaturateOnIntegerOverflow=on  InputSameDT=on
  data_out : Outport
  wires:
  Initial_Condition/1 -> switch1/1, switch2/1
  Reset/1 -> switch1/2, OR/1
  data_in/1 -> switch1/3
  Const_Zero/1 -> delay_up/1
  switch1/1 -> delay_down/1
  delay_up/1 -> OR/2
  OR/1 -> switch2/2
  delay_down/1 -> switch2/3
  switch2/1 -> data_out/1

== system gm_ModeS_ADI_Codegen/Detector/CalcCRC/crc24f/x22 ==
  data_in : Inport
  Reset : Inport  Port=2
  Const_Zero : Constant  Value=0  OutDataTypeStr=boolean
  Initial_Condition : Constant  Value=0.0  OutDataTypeStr=Inherit: Inherit via back propagation
  OR : Logic  Operator=OR
  delay_down : UnitDelay  SampleTime=-1
  delay_up : UnitDelay  InitialCondition=1  SampleTime=-1
  switch1 : Switch  SaturateOnIntegerOverflow=on  InputSameDT=on
  switch2 : Switch  SaturateOnIntegerOverflow=on  InputSameDT=on
  data_out : Outport
  wires:
  Initial_Condition/1 -> switch1/1, switch2/1
  Reset/1 -> switch1/2, OR/1
  data_in/1 -> switch1/3
  Const_Zero/1 -> delay_up/1
  switch1/1 -> delay_down/1
  delay_up/1 -> OR/2
  OR/1 -> switch2/2
  delay_down/1 -> switch2/3
  switch2/1 -> data_out/1

== system gm_ModeS_ADI_Codegen/Detector/CalcCRC/crc24f/x23 ==
  data_in : Inport
  Reset : Inport  Port=2
  Const_Zero : Constant  Value=0  OutDataTypeStr=boolean
  Initial_Condition : Constant  Value=0.0  OutDataTypeStr=Inherit: Inherit via back propagation
  OR : Logic  Operator=OR
  delay_down : UnitDelay  SampleTime=-1
  delay_up : UnitDelay  InitialCondition=1  SampleTime=-1
  switch1 : Switch  SaturateOnIntegerOverflow=on  InputSameDT=on
  switch2 : Switch  SaturateOnIntegerOverflow=on  InputSameDT=on
  data_out : Outport
  wires:
  Initial_Condition/1 -> switch1/1, switch2/1
  Reset/1 -> switch1/2, OR/1
  data_in/1 -> switch1/3
  Const_Zero/1 -> delay_up/1
  switch1/1 -> delay_down/1
  delay_up/1 -> OR/2
  OR/1 -> switch2/2
  delay_down/1 -> switch2/3
  switch2/1 -> data_out/1

== system gm_ModeS_ADI_Codegen/Detector/CalcCRC/crc24f/x3 ==
  data_in : Inport
  Reset : Inport  Port=2
  Const_Zero : Constant  Value=0  OutDataTypeStr=boolean
  Initial_Condition : Constant  Value=0.0  OutDataTypeStr=Inherit: Inherit via back propagation
  OR : Logic  Operator=OR
  delay_down : UnitDelay  SampleTime=-1
  delay_up : UnitDelay  InitialCondition=1  SampleTime=-1
  switch1 : Switch  SaturateOnIntegerOverflow=on  InputSameDT=on
  switch2 : Switch  SaturateOnIntegerOverflow=on  InputSameDT=on
  data_out : Outport
  wires:
  Initial_Condition/1 -> switch1/1, switch2/1
  Reset/1 -> switch1/2, OR/1
  data_in/1 -> switch1/3
  Const_Zero/1 -> delay_up/1
  switch1/1 -> delay_down/1
  delay_up/1 -> OR/2
  OR/1 -> switch2/2
  delay_down/1 -> switch2/3
  switch2/1 -> data_out/1

== system gm_ModeS_ADI_Codegen/Detector/CalcCRC/crc24f/x4 ==
  data_in : Inport
  Reset : Inport  Port=2
  Const_Zero : Constant  Value=0  OutDataTypeStr=boolean
  Initial_Condition : Constant  Value=0.0  OutDataTypeStr=Inherit: Inherit via back propagation
  OR : Logic  Operator=OR
  delay_down : UnitDelay  SampleTime=-1
  delay_up : UnitDelay  InitialCondition=1  SampleTime=-1
  switch1 : Switch  SaturateOnIntegerOverflow=on  InputSameDT=on
  switch2 : Switch  SaturateOnIntegerOverflow=on  InputSameDT=on
  data_out : Outport
  wires:
  Initial_Condition/1 -> switch1/1, switch2/1
  Reset/1 -> switch1/2, OR/1
  data_in/1 -> switch1/3
  Const_Zero/1 -> delay_up/1
  switch1/1 -> delay_down/1
  delay_up/1 -> OR/2
  OR/1 -> switch2/2
  delay_down/1 -> switch2/3
  switch2/1 -> data_out/1

== system gm_ModeS_ADI_Codegen/Detector/CalcCRC/crc24f/x5 ==
  data_in : Inport
  Reset : Inport  Port=2
  Const_Zero : Constant  Value=0  OutDataTypeStr=boolean
  Initial_Condition : Constant  Value=0.0  OutDataTypeStr=Inherit: Inherit via back propagation
  OR : Logic  Operator=OR
  delay_down : UnitDelay  SampleTime=-1
  delay_up : UnitDelay  InitialCondition=1  SampleTime=-1
  switch1 : Switch  SaturateOnIntegerOverflow=on  InputSameDT=on
  switch2 : Switch  SaturateOnIntegerOverflow=on  InputSameDT=on
  data_out : Outport
  wires:
  Initial_Condition/1 -> switch1/1, switch2/1
  Reset/1 -> switch1/2, OR/1
  data_in/1 -> switch1/3
  Const_Zero/1 -> delay_up/1
  switch1/1 -> delay_down/1
  delay_up/1 -> OR/2
  OR/1 -> switch2/2
  delay_down/1 -> switch2/3
  switch2/1 -> data_out/1

== system gm_ModeS_ADI_Codegen/Detector/CalcCRC/crc24f/x6 ==
  data_in : Inport
  Reset : Inport  Port=2
  Const_Zero : Constant  Value=0  OutDataTypeStr=boolean
  Initial_Condition : Constant  Value=0.0  OutDataTypeStr=Inherit: Inherit via back propagation
  OR : Logic  Operator=OR
  delay_down : UnitDelay  SampleTime=-1
  delay_up : UnitDelay  InitialCondition=1  SampleTime=-1
  switch1 : Switch  SaturateOnIntegerOverflow=on  InputSameDT=on
  switch2 : Switch  SaturateOnIntegerOverflow=on  InputSameDT=on
  data_out : Outport
  wires:
  Initial_Condition/1 -> switch1/1, switch2/1
  Reset/1 -> switch1/2, OR/1
  data_in/1 -> switch1/3
  Const_Zero/1 -> delay_up/1
  switch1/1 -> delay_down/1
  delay_up/1 -> OR/2
  OR/1 -> switch2/2
  delay_down/1 -> switch2/3
  switch2/1 -> data_out/1

== system gm_ModeS_ADI_Codegen/Detector/CalcCRC/crc24f/x7 ==
  data_in : Inport
  Reset : Inport  Port=2
  Const_Zero : Constant  Value=0  OutDataTypeStr=boolean
  Initial_Condition : Constant  Value=0.0  OutDataTypeStr=Inherit: Inherit via back propagation
  OR : Logic  Operator=OR
  delay_down : UnitDelay  SampleTime=-1
  delay_up : UnitDelay  InitialCondition=1  SampleTime=-1
  switch1 : Switch  SaturateOnIntegerOverflow=on  InputSameDT=on
  switch2 : Switch  SaturateOnIntegerOverflow=on  InputSameDT=on
  data_out : Outport
  wires:
  Initial_Condition/1 -> switch1/1, switch2/1
  Reset/1 -> switch1/2, OR/1
  data_in/1 -> switch1/3
  Const_Zero/1 -> delay_up/1
  switch1/1 -> delay_down/1
  delay_up/1 -> OR/2
  OR/1 -> switch2/2
  delay_down/1 -> switch2/3
  switch2/1 -> data_out/1

== system gm_ModeS_ADI_Codegen/Detector/CalcCRC/crc24f/x8 ==
  data_in : Inport
  Reset : Inport  Port=2
  Const_Zero : Constant  Value=0  OutDataTypeStr=boolean
  Initial_Condition : Constant  Value=0.0  OutDataTypeStr=Inherit: Inherit via back propagation
  OR : Logic  Operator=OR
  delay_down : UnitDelay  SampleTime=-1
  delay_up : UnitDelay  InitialCondition=1  SampleTime=-1
  switch1 : Switch  SaturateOnIntegerOverflow=on  InputSameDT=on
  switch2 : Switch  SaturateOnIntegerOverflow=on  InputSameDT=on
  data_out : Outport
  wires:
  Initial_Condition/1 -> switch1/1, switch2/1
  Reset/1 -> switch1/2, OR/1
  data_in/1 -> switch1/3
  Const_Zero/1 -> delay_up/1
  switch1/1 -> delay_down/1
  delay_up/1 -> OR/2
  OR/1 -> switch2/2
  delay_down/1 -> switch2/3
  switch2/1 -> data_out/1

== system gm_ModeS_ADI_Codegen/Detector/CalcCRC/crc24f/x9 ==
  data_in : Inport
  Reset : Inport  Port=2
  Const_Zero : Constant  Value=0  OutDataTypeStr=boolean
  Initial_Condition : Constant  Value=0.0  OutDataTypeStr=Inherit: Inherit via back propagation
  OR : Logic  Operator=OR
  delay_down : UnitDelay  SampleTime=-1
  delay_up : UnitDelay  InitialCondition=1  SampleTime=-1
  switch1 : Switch  SaturateOnIntegerOverflow=on  InputSameDT=on
  switch2 : Switch  SaturateOnIntegerOverflow=on  InputSameDT=on
  data_out : Outport
  wires:
  Initial_Condition/1 -> switch1/1, switch2/1
  Reset/1 -> switch1/2, OR/1
  data_in/1 -> switch1/3
  Const_Zero/1 -> delay_up/1
  switch1/1 -> delay_down/1
  delay_up/1 -> OR/2
  OR/1 -> switch2/2
  delay_down/1 -> switch2/3
  switch2/1 -> data_out/1

== stateflow chart gm_ModeS_ADI_Codegen/Detector/SyncAndControl/SyncAndControl ==
  settings: executeAtInitialization=1
  state SyncSearch
  state WaitForT0
    T0Delay++;
  state BitProcess
    SamplesIn++;
    Reset = 0;
  state ClearBP
    SamplesIn++;
  state EmptyReg
    CRCClocks++;
  (default) -> SyncSearch
  ClearBP -> SyncSearch [order 1] : [SamplesIn>100]
  SyncSearch -> WaitForT0 : [SyncCorr > 40*NoiseFloor]
      | {ActivateBP = 1;
      | maxSync = SyncCorr;
      | SamplesIn = 0;
      | T0Delay = 0;
      | Reset = 1;}
  WaitForT0 -> WaitForT0 [order 3]
  BitProcess -> WaitForT0 [order 2] : [SyncCorr > maxSync && SamplesIn < 50]
      | {Reset = 1;
      | SamplesIn = 0;
      | maxSync = SyncCorr;
      | T0Delay = 0;}
  WaitForT0 -> WaitForT0 [order 2] : [SyncCorr > maxSync]
      | {T0Delay = 0;
      | maxSync = SyncCorr;}
  WaitForT0 -> BitProcess [order 1] : [T0Delay>25]
  BitProcess -> BitProcess [order 3]
  ClearBP -> ClearBP [order 2]
  BitProcess -> EmptyReg [order 1] : [SamplesIn>=12.5*88]
      | {EmptyReg = 1;
      | CRCClocks = 0;}
  EmptyReg -> ClearBP [order 1] : [CRCClocks>=24*12.5]
      | {maxSync = 0;
      | ActivateBP = 0;
      | Reset = 0;
      | SamplesIn = 0;
      | EmptyReg = 0;}
  EmptyReg -> EmptyReg [order 2]
  data: NoiseFloor input; SyncCorr input; Reset output boolean =0; ActivateBP output boolean =0; EmptyReg output boolean =0; SamplesIn local uint16 =0; maxSync local fixdt(1,14,9) =0; CRCClocks local uint16 =0; T0Delay local uint8 =0
